simulink model "Lidar_System_FullStateOct25v2"  (Simulink 7.3)
settings: Solver=FixedStepDiscrete  StartTime=0.0  StopTime=inf  FixedStep=0.1  MaxStep=0.2  RelTol=1e-3
undefined symbols (not defined in the file): strel
libraries: dspmtrx3 x28, simulink x11, dspstat3 x10, vipstatistics x6, vipmorphops x6, dspindex x1
(part 1 of 3)
settings Model: Creator=gclayton  LastModifiedBy=wildcat
settings DebuggingCC: InheritedTsInSrcMsg=none
settings RTWCC: SystemTargetFile=rlnx.tlc  GenCodeOnly=on  TemplateMakefile=rlnx_ubuntu.tmf  Description=Linux Real-Time Target  ProcessScript=rlnx_make_rtw_hook
settings RTWCC: CustomInclude=|
  | /usr/local/include/opencv/
  | /usr/local/include/
settings CodeAppCC: GenerateComments=off  SimulinkBlockComments=off
settings STFCustomTargetCC: ModelReferenceCompliant=off  MatFileLogging=on  SystemTargetFile=rlnx.tlc
settings GRTTargetCC: ModelReferenceCompliant=off  ParMdlRefBuildCompliant=off  CompOptLevelCompliant=off  ExtModeMexFile=noextcomm
settings CustomProperty: DataType=string  Value="-lm -ldl /usr/local/lib/libopencv_highgui.so.2.4 /usr/local/lib/libopencv_core.so.2.4 /usr/local/lib/libopencv_imgproc.so.2.4  -lc_urg -lc_urg_connection -lc_urg_system -lphidget21 -llcm"
settings EnumStrPairs: String=PC

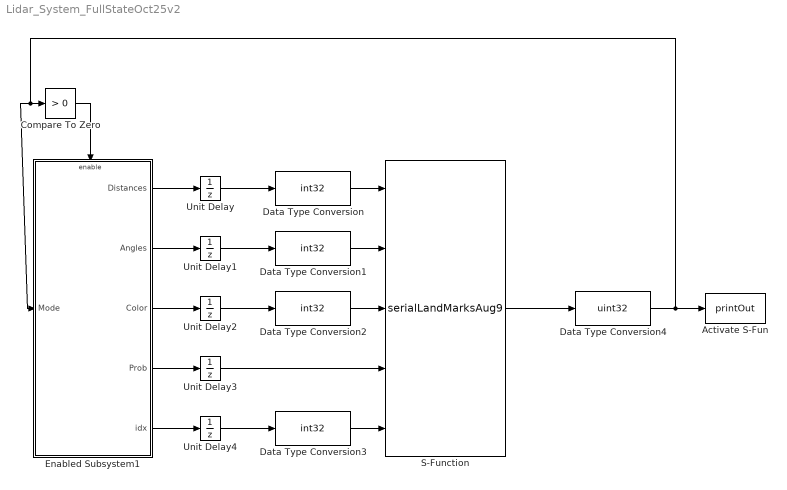
== system Lidar_System_FullStateOct25v2 ==
  Activate S-Fun : S-Function  FunctionName=printOut  EnableBusSupport=off
  Compare To Zero : simulink/Logic and Bit Operations/Compare To Zero  SystemSampleTime=-1  relop=>  LogicOutDataTypeMode=uint8  ZeroCross=off
  Data Type Conversion{,1..3} (4 alike) : DataTypeConversion  OutDataTypeMode=int32  OutDataType=fixdt(1, 16)  OutScaling=2^0  OutDataTypeStr=int32
  Data Type Conversion4 : DataTypeConversion  OutDataTypeMode=uint32  OutDataType=fixdt(1, 16)  OutScaling=2^0  OutDataTypeStr=uint32
  Enabled Subsystem1 : Subsystem  TreatAsAtomicUnit=on
  S-Function : S-Function  FunctionName=serialLandMarksAug9  EnableBusSupport=off
  Unit Delay : UnitDelay  X0=zeros(1,12)  SampleTime=-1
  Unit Delay1 : UnitDelay  X0=zeros(1,12)  SampleTime=-1
  Unit Delay2 : UnitDelay  X0=zeros(4,1)  SampleTime=-1
  Unit Delay3 : UnitDelay  X0=zeros(4,1)  SampleTime=-1
  Unit Delay4 : UnitDelay  X0=zeros(4,1)  SampleTime=-1
  wires:
  Compare To Zero/1 -> Enabled Subsystem1/Enable
  Data Type Conversion4/1 -> Activate S-Fun/1, Compare To Zero/1, Enabled Subsystem1/1(Mode)
  S-Function/1 -> Data Type Conversion4/1
  Enabled Subsystem1/2(Angles) -> Unit Delay1/1
  Enabled Subsystem1/1(Distances) -> Unit Delay/1
  Enabled Subsystem1/3(Color) -> Unit Delay2/1
  Enabled Subsystem1/4(Prob) -> Unit Delay3/1
  Enabled Subsystem1/5(idx) -> Unit Delay4/1
  Unit Delay/1 -> Data Type Conversion/1
  Unit Delay1/1 -> Data Type Conversion1/1
  Unit Delay2/1 -> Data Type Conversion2/1
  Unit Delay4/1 -> Data Type Conversion3/1
  Data Type Conversion/1 -> S-Function/1
  Data Type Conversion1/1 -> S-Function/2
  Data Type Conversion2/1 -> S-Function/3
  Unit Delay3/1 -> S-Function/4
  Data Type Conversion3/1 -> S-Function/5

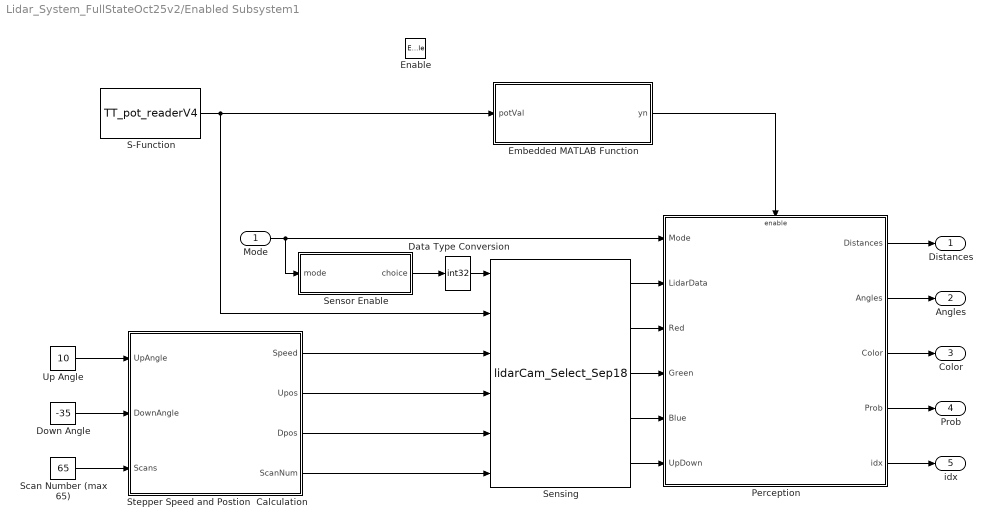
== system Lidar_System_FullStateOct25v2/Enabled Subsystem1 ==
  Mode : Inport  OutDataType=fixdt(1, 16)  OutScaling=2^0
  Enable : EnablePort
  Data Type Conversion : DataTypeConversion  OutDataTypeMode=int32  OutDataType=fixdt(1, 16)  OutScaling=2^0  OutDataTypeStr=int32
  Down Angle : Constant  Value=-35  OutDataType=fixdt(1, 16)  OutScaling=2^0
  Embedded MATLAB Function : Stateflow chart
  Perception : Subsystem  TreatAsAtomicUnit=on
  S-Function : S-Function  FunctionName=TT_pot_readerV4  EnableBusSupport=off
  Scan Number (max 65) : Constant  Value=65  OutDataType=fixdt(1, 16)  OutScaling=2^0
  Sensing : S-Function  FunctionName=lidarCam_Select_Sep18  EnableBusSupport=off
  Sensor Enable : Stateflow chart
  Stepper Speed and Postion  Calculation : Stateflow chart
  Up Angle : Constant  Value=10  OutDataType=fixdt(1, 16)  OutScaling=2^0
  Distances : Outport  OutDataType=fixdt(1, 16)  OutScaling=2^0
  Angles : Outport  Port=2  OutDataType=fixdt(1, 16)  OutScaling=2^0
  Color : Outport  Port=3  OutDataType=fixdt(1, 16)  OutScaling=2^0
  Prob : Outport  Port=4  OutDataType=fixdt(1, 16)  OutScaling=2^0
  idx : Outport  Port=5  OutDataType=fixdt(1, 16)  OutScaling=2^0
  wires:
  Embedded MATLAB Function/1(yn) -> Perception/Enable
  Sensing/1 -> Perception/2(LidarData)
  Sensing/5 -> Perception/6(UpDown)
  Sensing/2 -> Perception/3(Red)
  Sensing/3 -> Perception/4(Green)
  Sensing/4 -> Perception/5(Blue)
  Mode/1 -> Perception/1(Mode), Sensor Enable/1(mode)
  Down Angle/1 -> Stepper Speed and Postion  Calculation/2(DownAngle)
  Up Angle/1 -> Stepper Speed and Postion  Calculation/1(UpAngle)
  Scan Number (max 65)/1 -> Stepper Speed and Postion  Calculation/3(Scans)
  Stepper Speed and Postion  Calculation/1(Speed) -> Sensing/3
  Stepper Speed and Postion  Calculation/2(Upos) -> Sensing/4
  Stepper Speed and Postion  Calculation/3(Dpos) -> Sensing/5
  Stepper Speed and Postion  Calculation/4(ScanNum) -> Sensing/6
  S-Function/1 -> Embedded MATLAB Function/1(potVal), Sensing/2
  Sensor Enable/1(choice) -> Data Type Conversion/1
  Data Type Conversion/1 -> Sensing/1
  Perception/1(Distances) -> Distances/1
  Perception/2(Angles) -> Angles/1
  Perception/3(Color) -> Color/1
  Perception/4(Prob) -> Prob/1
  Perception/5(idx) -> idx/1

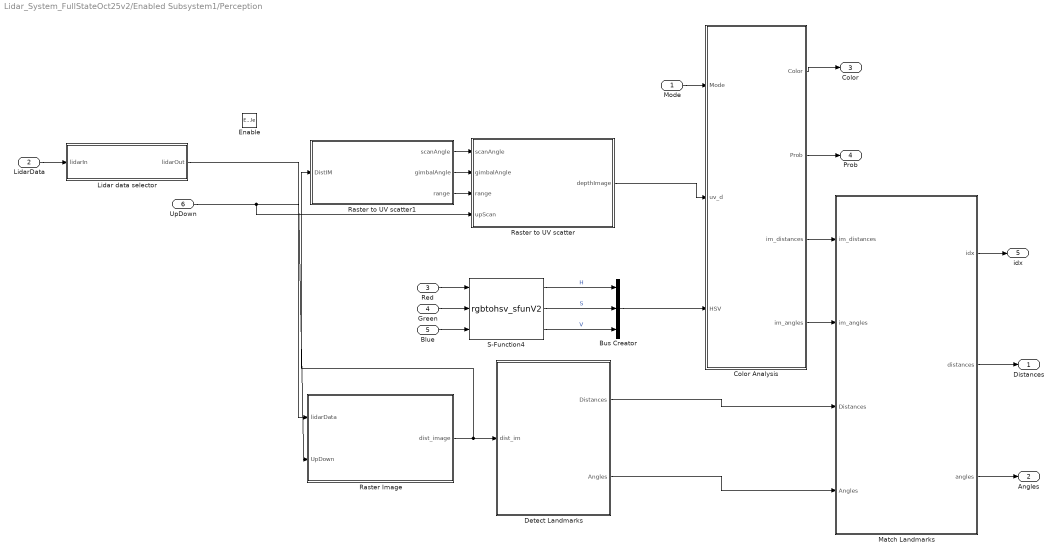
== system Lidar_System_FullStateOct25v2/Enabled Subsystem1/Perception ==
  Mode : Inport  OutDataType=fixdt(1, 16)  OutScaling=2^0
  LidarData : Inport  Port=2  OutDataType=fixdt(1, 16)  OutScaling=2^0
  Red : Inport  Port=3  OutDataType=fixdt(1, 16)  OutScaling=2^0
  Green : Inport  Port=4  OutDataType=fixdt(1, 16)  OutScaling=2^0
  Blue : Inport  Port=5  OutDataType=fixdt(1, 16)  OutScaling=2^0
  UpDown : Inport  Port=6  OutDataType=fixdt(1, 16)  OutScaling=2^0
  Enable : EnablePort
  Bus Creator : BusCreator  Inputs=3
  Color Analysis : Subsystem
  Detect Landmarks : Subsystem
  Lidar data selector : Stateflow chart
  Match Landmarks : Stateflow chart
  Raster Image : Stateflow chart
  Raster to UV scatter : Stateflow chart
  Raster to UV scatter1 : Stateflow chart
  S-Function4 : S-Function  FunctionName=rgbtohsv_sfunV2  EnableBusSupport=off
  Distances : Outport  OutDataType=fixdt(1, 16)  OutScaling=2^0
  Angles : Outport  Port=2  OutDataType=fixdt(1, 16)  OutScaling=2^0
  Color : Outport  Port=3  OutDataType=fixdt(1, 16)  OutScaling=2^0
  Prob : Outport  Port=4  OutDataType=fixdt(1, 16)  OutScaling=2^0
  idx : Outport  Port=5  OutDataType=fixdt(1, 16)  OutScaling=2^0
  wires:
  Lidar data selector/1(lidarOut) -> Raster Image/1(lidarData)
  UpDown/1 -> Raster Image/2(UpDown), Raster to UV scatter/4(upScan)
  Red/1 -> S-Function4/1
  Green/1 -> S-Function4/2
  Blue/1 -> S-Function4/3
  LidarData/1 -> Lidar data selector/1(lidarIn)
  S-Function4/1 -> Bus Creator/1  "H"
  S-Function4/2 -> Bus Creator/2  "S"
  S-Function4/3 -> Bus Creator/3  "V"
  Bus Creator/1 -> Color Analysis/3(HSV)
  Raster to UV scatter/1(depthImage) -> Color Analysis/2(uv_d)
  Mode/1 -> Color Analysis/1(Mode)
  Color Analysis/2(Prob) -> Prob/1
  Color Analysis/1(Color) -> Color/1
  Color Analysis/3(im_distances) -> Match Landmarks/1(im_distances)
  Color Analysis/4(im_angles) -> Match Landmarks/2(im_angles)
  Detect Landmarks/1(Distances) -> Match Landmarks/3(Distances)
  Detect Landmarks/2(Angles) -> Match Landmarks/4(Angles)
  Raster Image/1(dist_image) -> Detect Landmarks/1(dist_im), Raster to UV scatter1/1(DistIM)
  Raster to UV scatter1/1(scanAngle) -> Raster to UV scatter/1(scanAngle)
  Raster to UV scatter1/2(gimbalAngle) -> Raster to UV scatter/2(gimbalAngle)
  Raster to UV scatter1/3(range) -> Raster to UV scatter/3(range)
  Match Landmarks/1(idx) -> idx/1
  Match Landmarks/2(distances) -> Distances/1
  Match Landmarks/3(angles) -> Angles/1

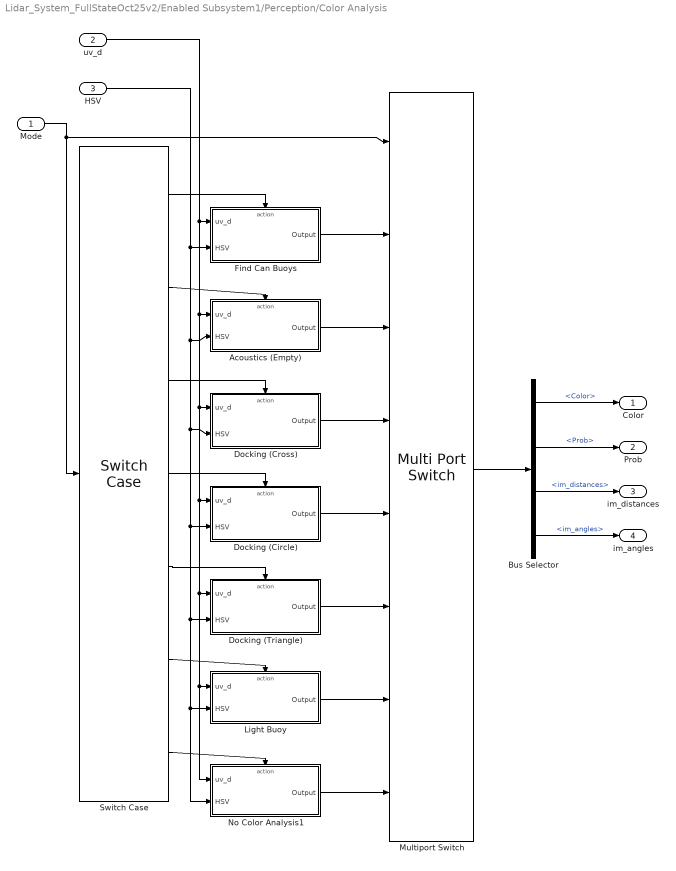
== system Lidar_System_FullStateOct25v2/Enabled Subsystem1/Perception/Color Analysis ==
  Mode : Inport  OutDataType=fixdt(1, 16)  OutScaling=2^0
  uv_d : Inport  Port=2  OutDataType=fixdt(1, 16)  OutScaling=2^0
  HSV : Inport  Port=3  OutDataType=fixdt(1, 16)  OutScaling=2^0
  Acoustics (Empty) : Subsystem  TreatAsAtomicUnit=on
  Bus Selector : BusSelector  OutputSignals=Color,Prob,im_distances,im_angles
  Docking (Circle) : Subsystem  TreatAsAtomicUnit=on
  Docking (Cross) : Subsystem  TreatAsAtomicUnit=on
  Docking (Triangle) : Subsystem  TreatAsAtomicUnit=on
  Find Can Buoys : Subsystem  TreatAsAtomicUnit=on
  Light Buoy : Subsystem  TreatAsAtomicUnit=on
  Multiport Switch : MultiPortSwitch  Inputs=7  OutDataType=fixdt(1, 16)  OutScaling=2^0
  No Color Analysis1 : Subsystem  TreatAsAtomicUnit=on
  Switch Case : SwitchCase  CaseConditions={1,2,3,4,5,6}
  Color : Outport  OutDataType=fixdt(1, 16)  OutScaling=2^0
  Prob : Outport  Port=2  OutDataType=fixdt(1, 16)  OutScaling=2^0
  im_distances : Outport  Port=3  OutDataType=fixdt(1, 16)  OutScaling=2^0
  im_angles : Outport  Port=4  OutDataType=fixdt(1, 16)  OutScaling=2^0
  wires:
  Switch Case/1 -> Find Can Buoys/Action
  Mode/1 -> Switch Case/1, Multiport Switch/1
  Switch Case/2 -> Acoustics (Empty)/Action
  Switch Case/3 -> Docking (Cross)/Action
  Find Can Buoys/1(Output) -> Multiport Switch/2
  Docking (Cross)/1(Output) -> Multiport Switch/4
  Docking (Circle)/1(Output) -> Multiport Switch/5
  uv_d/1 -> Docking (Cross)/1(uv_d), Docking (Circle)/1(uv_d), Docking (Triangle)/1(uv_d), Light Buoy/1(uv_d), No Color Analysis1/1(uv_d), Acoustics (Empty)/1(uv_d), Find Can Buoys/1(uv_d)
  HSV/1 -> Docking (Cross)/2(HSV), Docking (Circle)/2(HSV), Docking (Triangle)/2(HSV), Light Buoy/2(HSV), No Color Analysis1/2(HSV), Acoustics (Empty)/2(HSV), Find Can Buoys/2(HSV)
  Acoustics (Empty)/1(Output) -> Multiport Switch/3
  Bus Selector/1 -> Color/1  "<Color>"
  Bus Selector/2 -> Prob/1  "<Prob>"
  Bus Selector/3 -> im_distances/1  "<im_distances>"
  Bus Selector/4 -> im_angles/1  "<im_angles>"
  Switch Case/4 -> Docking (Circle)/Action
  Switch Case/7 -> No Color Analysis1/Action
  Switch Case/5 -> Docking (Triangle)/Action
  Switch Case/6 -> Light Buoy/Action
  Docking (Triangle)/1(Output) -> Multiport Switch/6
  Light Buoy/1(Output) -> Multiport Switch/7
  No Color Analysis1/1(Output) -> Multiport Switch/8
  Multiport Switch/1 -> Bus Selector/1

== system Lidar_System_FullStateOct25v2/Enabled Subsystem1/Perception/Detect Landmarks ==
  dist_im : Inport  OutDataType=fixdt(1, 16)  OutScaling=2^0
  Blob Analysis : vipstatistics/Blob Analysis  DialogController=vipDDGCreate  DialogControllerArgs=DataTag15  area=off  centroid=on  bBox=on  majorAxis=off  minorAxis=off  angle=off  eccentricity=off  equivDiameterSq=off  extent=off  perimeter=off  maxBlobs=12  warnIfNumBlobsExceeded=on  isCount=off  useMinArea=on  minArea=30  useMaxArea=off  maxArea=intmax('uint32')  excludeBorderBlob=on  outDT=double  isOutVarDim=off  isFill=on  fillValues=-1  conn=8  isLabel=off  outputMode=Binary point scaling  outputWordLength=32  outputFracLength=16  firstCoeffMode=Binary point scaling  firstCoeffWordLength=16  firstCoeffFracLength=14  secondCoeffMode=Binary point scaling  secondCoeffWordLength=32  secondCoeffFracLength=16  accumMode=Binary point scaling  accumWordLength=32  accumFracLength=0  prodOutputMode=Binary point scaling  prodOutputWordLength=32  prodOutputFracLength=16  roundingMode=Floor  overflowMode=off
  Closing : vipmorphops/Closing  nhoodsrc=Specify via dialog  strel=strel('rectangle',[5 7])
  Embedded MATLAB Function1 : Stateflow chart
  Logical Operator : Logic  AllPortsSameDT=off  OutDataTypeMode=boolean  LogicDataType=fixdt(0, 8)  OutDataTypeStr=boolean
  Max Thresh : simulink/Logic and Bit Operations/Compare To Constant  SystemSampleTime=-1  relop=<=  const=10000  LogicOutDataTypeMode=boolean  ZeroCross=off
  Min Thresh (removes pontoons) : simulink/Logic and Bit Operations/Compare To Constant  SystemSampleTime=-1  relop=>  const=5000  LogicOutDataTypeMode=boolean  ZeroCross=off
  Distances : Outport  OutDataType=fixdt(1, 16)  OutScaling=2^0
  Angles : Outport  Port=2  OutDataType=fixdt(1, 16)  OutScaling=2^0
  wires:
  Max Thresh/1 -> Logical Operator/1
  Min Thresh (removes pontoons)/1 -> Logical Operator/2
  dist_im/1 -> Max Thresh/1, Min Thresh (removes pontoons)/1, Embedded MATLAB Function1/4(dist_im)
  Embedded MATLAB Function1/1(Distances) -> Distances/1
  Embedded MATLAB Function1/2(Angles) -> Angles/1
  Logical Operator/1 -> Closing/1, Embedded MATLAB Function1/3(BW)
  Closing/1 -> Blob Analysis/1
  Blob Analysis/1 -> Embedded MATLAB Function1/1(centroid)
  Blob Analysis/2 -> Embedded MATLAB Function1/2(bbox)

== system Lidar_System_FullStateOct25v2/Enabled Subsystem1/Perception/Color Analysis/Acoustics (Empty) ==
  uv_d : Inport  OutDataType=fixdt(1, 16)  OutScaling=2^0
  HSV : Inport  Port=2  OutDataType=fixdt(1, 16)  OutScaling=2^0
  Action Port : ActionPort  ActionType=case
  Bus Creator : BusCreator
  Constant{,1..3} (4 alike) : Constant  Value=zeros(4,1)  OutDataType=fixdt(1, 16)  OutScaling=2^0
  Terminator : Terminator
  Terminator1 : Terminator
  Output : Outport  OutDataType=fixdt(1, 16)  OutScaling=2^0
  wires:
  uv_d/1 -> Terminator/1
  HSV/1 -> Terminator1/1
  Bus Creator/1 -> Output/1
  Constant3/1 -> Bus Creator/4  "im_angles"
  Constant2/1 -> Bus Creator/3  "im_distances"
  Constant1/1 -> Bus Creator/2  "Prob"
  Constant/1 -> Bus Creator/1  "Color"

== system Lidar_System_FullStateOct25v2/Enabled Subsystem1/Perception/Color Analysis/Docking (Circle) ==
  uv_d : Inport  OutDataType=fixdt(1, 16)  OutScaling=2^0
  HSV : Inport  Port=2  OutDataType=fixdt(1, 16)  OutScaling=2^0
  Action Port : ActionPort  ActionType=case
  Bus Creator : BusCreator
  Bus Selector : BusSelector  OutputSignals=H,S,V
  Constant : Constant  Value=zeros(4,1)  OutDataType=fixdt(1, 16)  OutScaling=2^0
  Constant1 : Constant  Value=zeros(4,1)  OutDataType=fixdt(1, 16)  OutScaling=2^0
  Constant4 : Constant  Value=2  OutDataType=fixdt(1, 16)  OutScaling=2^0
  Docking1 : Subsystem
  Output : Outport  OutDataType=fixdt(1, 16)  OutScaling=2^0
  wires:
  Constant/1 -> Bus Creator/1  "Color"
  Constant1/1 -> Bus Creator/2  "Prob"
  Docking1/1(Distances) -> Bus Creator/3  "im_distances"
  Docking1/2(Angles) -> Bus Creator/4  "im_angles"
  Bus Creator/1 -> Output/1
  Constant4/1 -> Docking1/1(Target)
  Bus Selector/1 -> Docking1/2(H)  "<H>"
  Bus Selector/2 -> Docking1/3(S)  "<S>"
  Bus Selector/3 -> Docking1/4(V)  "<V>"
  HSV/1 -> Bus Selector/1
  uv_d/1 -> Docking1/5(uv_d)

== system Lidar_System_FullStateOct25v2/Enabled Subsystem1/Perception/Color Analysis/Docking (Cross) ==
  uv_d : Inport  OutDataType=fixdt(1, 16)  OutScaling=2^0
  HSV : Inport  Port=2  OutDataType=fixdt(1, 16)  OutScaling=2^0
  Action Port : ActionPort  ActionType=case
  Bus Creator : BusCreator
  Bus Selector : BusSelector  OutputSignals=H,S,V
  Constant : Constant  Value=zeros(4,1)  OutDataType=fixdt(1, 16)  OutScaling=2^0
  Constant1 : Constant  Value=zeros(4,1)  OutDataType=fixdt(1, 16)  OutScaling=2^0
  Constant4 : Constant  OutDataType=fixdt(1, 16)  OutScaling=2^0
  Docking1 : Subsystem
  Output : Outport  OutDataType=fixdt(1, 16)  OutScaling=2^0
  wires:
  uv_d/1 -> Docking1/5(uv_d)
  HSV/1 -> Bus Selector/1
  Bus Selector/3 -> Docking1/4(V)  "<V>"
  Bus Selector/2 -> Docking1/3(S)  "<S>"
  Bus Selector/1 -> Docking1/2(H)  "<H>"
  Constant4/1 -> Docking1/1(Target)
  Bus Creator/1 -> Output/1
  Docking1/2(Angles) -> Bus Creator/4  "im_angles"
  Docking1/1(Distances) -> Bus Creator/3  "im_distances"
  Constant1/1 -> Bus Creator/2  "Prob"
  Constant/1 -> Bus Creator/1  "Color"

== system Lidar_System_FullStateOct25v2/Enabled Subsystem1/Perception/Color Analysis/Docking (Triangle) ==
  uv_d : Inport  OutDataType=fixdt(1, 16)  OutScaling=2^0
  HSV : Inport  Port=2  OutDataType=fixdt(1, 16)  OutScaling=2^0
  Action Port : ActionPort  ActionType=case
  Bus Creator : BusCreator
  Bus Selector : BusSelector  OutputSignals=H,S,V
  Constant : Constant  Value=zeros(4,1)  OutDataType=fixdt(1, 16)  OutScaling=2^0
  Constant1 : Constant  Value=zeros(4,1)  OutDataType=fixdt(1, 16)  OutScaling=2^0
  Constant4 : Constant  Value=3  OutDataType=fixdt(1, 16)  OutScaling=2^0
  Docking1 : Subsystem
  Output : Outport  OutDataType=fixdt(1, 16)  OutScaling=2^0
  wires:
  uv_d/1 -> Docking1/5(uv_d)
  HSV/1 -> Bus Selector/1
  Bus Selector/3 -> Docking1/4(V)  "<V>"
  Bus Selector/2 -> Docking1/3(S)  "<S>"
  Bus Selector/1 -> Docking1/2(H)  "<H>"
  Constant4/1 -> Docking1/1(Target)
  Bus Creator/1 -> Output/1
  Docking1/2(Angles) -> Bus Creator/4  "im_angles"
  Docking1/1(Distances) -> Bus Creator/3  "im_distances"
  Constant1/1 -> Bus Creator/2  "Prob"
  Constant/1 -> Bus Creator/1  "Color"

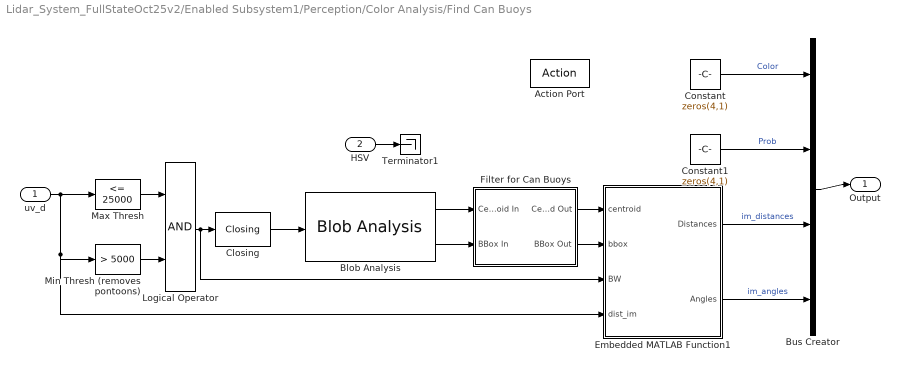
== system Lidar_System_FullStateOct25v2/Enabled Subsystem1/Perception/Color Analysis/Find Can Buoys ==
  uv_d : Inport  OutDataType=fixdt(1, 16)  OutScaling=2^0
  HSV : Inport  Port=2  OutDataType=fixdt(1, 16)  OutScaling=2^0
  Action Port : ActionPort  ActionType=case
  Blob Analysis : vipstatistics/Blob Analysis  DialogController=vipDDGCreate  DialogControllerArgs=DataTag12  area=off  centroid=on  bBox=on  majorAxis=off  minorAxis=off  angle=off  eccentricity=off  equivDiameterSq=off  extent=off  perimeter=off  maxBlobs=12  warnIfNumBlobsExceeded=on  isCount=off  useMinArea=on  minArea=30  useMaxArea=off  maxArea=intmax('uint32')  excludeBorderBlob=on  outDT=double  isOutVarDim=off  isFill=on  fillValues=-1  conn=8  isLabel=off  outputMode=Binary point scaling  outputWordLength=32  outputFracLength=16  firstCoeffMode=Binary point scaling  firstCoeffWordLength=16  firstCoeffFracLength=14  secondCoeffMode=Binary point scaling  secondCoeffWordLength=32  secondCoeffFracLength=16  accumMode=Binary point scaling  accumWordLength=32  accumFracLength=0  prodOutputMode=Binary point scaling  prodOutputWordLength=32  prodOutputFracLength=16  roundingMode=Floor  overflowMode=off
  Bus Creator : BusCreator
  Closing : vipmorphops/Closing  nhoodsrc=Specify via dialog  strel=strel('rectangle',[5 7])
  Constant : Constant  Value=zeros(4,1)  OutDataType=fixdt(1, 16)  OutScaling=2^0
  Constant1 : Constant  Value=zeros(4,1)  OutDataType=fixdt(1, 16)  OutScaling=2^0
  Embedded MATLAB Function1 : Stateflow chart
  Filter for Can Buoys : Subsystem
  Logical Operator : Logic  AllPortsSameDT=off  OutDataTypeMode=boolean  LogicDataType=fixdt(0, 8)  OutDataTypeStr=boolean
  Max Thresh : simulink/Logic and Bit Operations/Compare To Constant  SystemSampleTime=-1  relop=<=  const=25000  LogicOutDataTypeMode=boolean  ZeroCross=off
  Min Thresh (removes pontoons) : simulink/Logic and Bit Operations/Compare To Constant  SystemSampleTime=-1  relop=>  const=5000  LogicOutDataTypeMode=boolean  ZeroCross=off
  Terminator1 : Terminator
  Output : Outport  OutDataType=fixdt(1, 16)  OutScaling=2^0
  wires:
  Constant/1 -> Bus Creator/1  "Color"
  Constant1/1 -> Bus Creator/2  "Prob"
  Embedded MATLAB Function1/1(Distances) -> Bus Creator/3  "im_distances"
  Embedded MATLAB Function1/2(Angles) -> Bus Creator/4  "im_angles"
  Bus Creator/1 -> Output/1
  HSV/1 -> Terminator1/1
  Max Thresh/1 -> Logical Operator/1
  Min Thresh (removes pontoons)/1 -> Logical Operator/2
  Logical Operator/1 -> Closing/1, Embedded MATLAB Function1/3(BW)
  Closing/1 -> Blob Analysis/1
  uv_d/1 -> Max Thresh/1, Min Thresh (removes pontoons)/1, Embedded MATLAB Function1/4(dist_im)
  Blob Analysis/1 -> Filter for Can Buoys/1(Centroid In)
  Blob Analysis/2 -> Filter for Can Buoys/2(BBox In)
  Filter for Can Buoys/1(Centroid Out) -> Embedded MATLAB Function1/1(centroid)
  Filter for Can Buoys/2(BBox Out) -> Embedded MATLAB Function1/2(bbox)

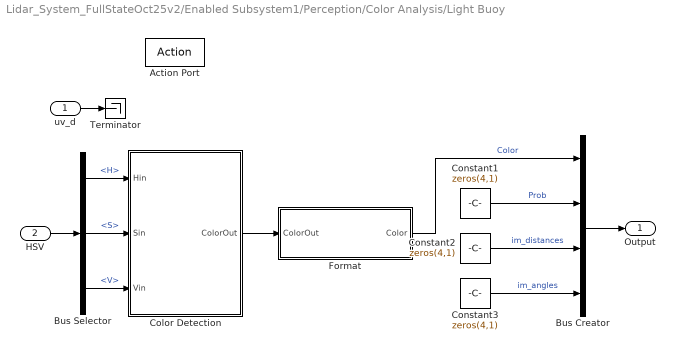
== system Lidar_System_FullStateOct25v2/Enabled Subsystem1/Perception/Color Analysis/Light Buoy ==
  uv_d : Inport  OutDataType=fixdt(1, 16)  OutScaling=2^0
  HSV : Inport  Port=2  OutDataType=fixdt(1, 16)  OutScaling=2^0
  Action Port : ActionPort  ActionType=case
  Bus Creator : BusCreator
  Bus Selector : BusSelector  OutputSignals=H,S,V
  Color Detection : Subsystem
  Constant1 : Constant  Value=zeros(4,1)  OutDataType=fixdt(1, 16)  OutScaling=2^0
  Constant2 : Constant  Value=zeros(4,1)  OutDataType=fixdt(1, 16)  OutScaling=2^0
  Constant3 : Constant  Value=zeros(4,1)  OutDataType=fixdt(1, 16)  OutScaling=2^0
  Format : Stateflow chart
  Terminator : Terminator
  Output : Outport  OutDataType=fixdt(1, 16)  OutScaling=2^0
  wires:
  Color Detection/1(ColorOut) -> Format/1(ColorOut)
  Bus Selector/3 -> Color Detection/3(Vin)  "<V>"
  Bus Selector/2 -> Color Detection/2(Sin)  "<S>"
  Bus Selector/1 -> Color Detection/1(Hin)  "<H>"
  HSV/1 -> Bus Selector/1
  uv_d/1 -> Terminator/1
  Bus Creator/1 -> Output/1
  Constant3/1 -> Bus Creator/4  "im_angles"
  Constant2/1 -> Bus Creator/3  "im_distances"
  Constant1/1 -> Bus Creator/2  "Prob"
  Format/1(Color) -> Bus Creator/1  "Color"

== system Lidar_System_FullStateOct25v2/Enabled Subsystem1/Perception/Color Analysis/No Color Analysis1 ==
  uv_d : Inport  OutDataType=fixdt(1, 16)  OutScaling=2^0
  HSV : Inport  Port=2  OutDataType=fixdt(1, 16)  OutScaling=2^0
  Action Port : ActionPort  ActionType=default
  Bus Creator : BusCreator
  Constant{,1..3} (4 alike) : Constant  Value=zeros(4,1)  OutDataType=fixdt(1, 16)  OutScaling=2^0
  Terminator : Terminator
  Terminator1 : Terminator
  Output : Outport  OutDataType=fixdt(1, 16)  OutScaling=2^0
  wires:
  Constant/1 -> Bus Creator/1  "Color"
  Constant1/1 -> Bus Creator/2  "Prob"
  Constant2/1 -> Bus Creator/3  "im_distances"
  Constant3/1 -> Bus Creator/4  "im_angles"
  Bus Creator/1 -> Output/1
  HSV/1 -> Terminator1/1
  uv_d/1 -> Terminator/1

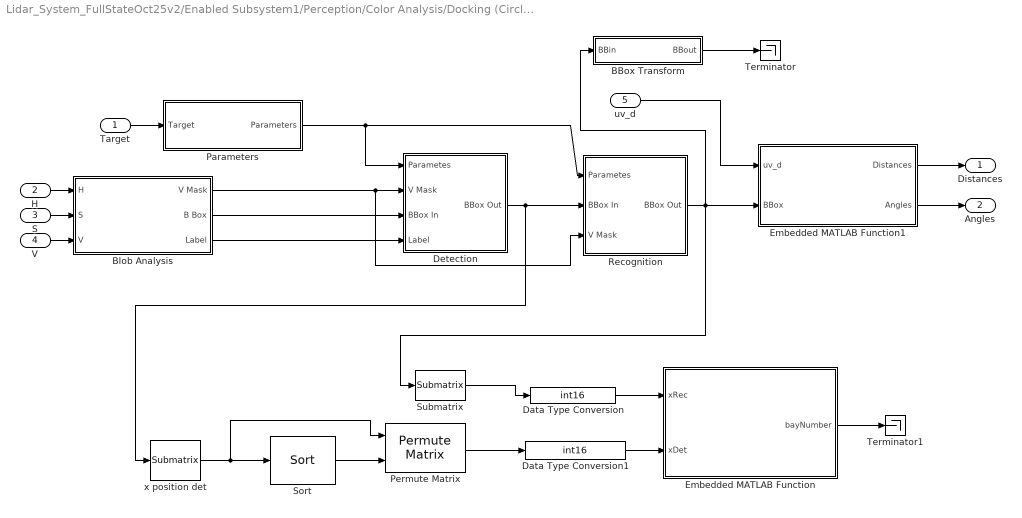
== system Lidar_System_FullStateOct25v2/Enabled Subsystem1/Perception/Color Analysis/Docking (Circle)/Docking1 ==
  Target : Inport
  H : Inport  Port=2
  S : Inport  Port=3
  V : Inport  Port=4
  uv_d : Inport  Port=5
  BBox Transform : Stateflow chart
  Blob Analysis : Subsystem
  Data Type Conversion : DataTypeConversion  OutDataTypeMode=int16  OutDataType=fixdt(1, 16)  OutScaling=2^0  OutDataTypeStr=int16
  Data Type Conversion1 : DataTypeConversion  OutDataTypeMode=int16  OutDataType=fixdt(1, 16)  OutScaling=2^0  OutDataTypeStr=int16
  Detection : Subsystem
  Embedded MATLAB Function : Stateflow chart
  Embedded MATLAB Function1 : Stateflow chart
  Parameters : Subsystem
  Permute Matrix : dspmtrx3/Permute Matrix  mode=Rows  ZeroOneIdxMode=One-based  errmode=Clip index  checkDims=off
  Recognition : Subsystem
  Sort : dspstat3/Sort  DialogController=dspDDGCreate  DialogControllerArgs=DataTag3  otype=Index  dir=Ascending  sortAlg=Quick sort  roundingMode=Floor  overflowMode=off
  Submatrix : dspmtrx3/Submatrix  RowSpan=Range of rows  RowStartMode=First  RowStartIndex=1  RowEndMode=Last  RowEndIndex=1  ColSpan=One column  ColStartMode=First  ColStartIndex=1  ColEndMode=Last  ColEndIndex=1
  Terminator : Terminator
  Terminator1 : Terminator
  x position det : dspmtrx3/Submatrix  RowSpan=Range of rows  RowStartMode=First  RowStartIndex=1  RowEndMode=Last  RowEndIndex=1  ColSpan=One column  ColStartMode=First  ColStartIndex=1  ColEndMode=Last  ColEndIndex=1
  Distances : Outport
  Angles : Outport  Port=2
  wires:
  Parameters/1(Parameters) -> Detection/1(Parametes), Recognition/1(Parametes)
  Blob Analysis/1(V Mask) -> Detection/2(V Mask), Recognition/3(V Mask)
  Blob Analysis/2(B Box) -> Detection/3(BBox In)
  Blob Analysis/3(Label) -> Detection/4(Label)
  Detection/1(BBox Out) -> Recognition/2(BBox In), x position det/1
  x position det/1 -> Sort/1, Permute Matrix/1
  Sort/1 -> Permute Matrix/2
  Submatrix/1 -> Data Type Conversion/1
  Permute Matrix/1 -> Data Type Conversion1/1
  Data Type Conversion/1 -> Embedded MATLAB Function/1(xRec)
  Data Type Conversion1/1 -> Embedded MATLAB Function/2(xDet)
  Recognition/1(BBox Out) -> Submatrix/1, Embedded MATLAB Function1/2(BBox), BBox Transform/1(BBin)
  Embedded MATLAB Function/1(bayNumber) -> Terminator1/1
  uv_d/1 -> Embedded MATLAB Function1/1(uv_d)
  Embedded MATLAB Function1/1(Distances) -> Distances/1
  H/1 -> Blob Analysis/1(H)
  S/1 -> Blob Analysis/2(S)
  V/1 -> Blob Analysis/3(V)
  Target/1 -> Parameters/1(Target)
  BBox Transform/1(BBout) -> Terminator/1
  Embedded MATLAB Function1/2(Angles) -> Angles/1

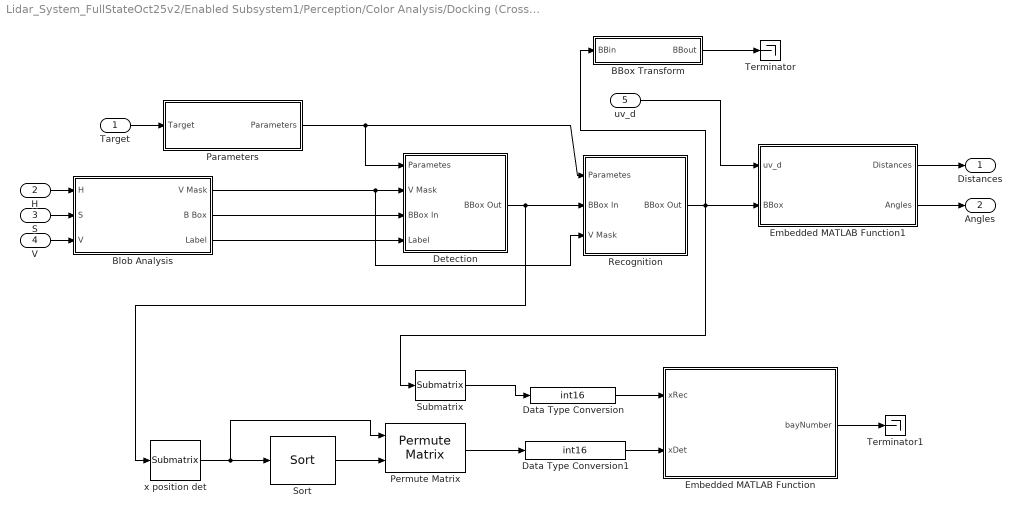
== system Lidar_System_FullStateOct25v2/Enabled Subsystem1/Perception/Color Analysis/Docking (Cross)/Docking1 ==
  Target : Inport
  H : Inport  Port=2
  S : Inport  Port=3
  V : Inport  Port=4
  uv_d : Inport  Port=5
  BBox Transform : Stateflow chart
  Blob Analysis : Subsystem
  Data Type Conversion : DataTypeConversion  OutDataTypeMode=int16  OutDataType=fixdt(1, 16)  OutScaling=2^0  OutDataTypeStr=int16
  Data Type Conversion1 : DataTypeConversion  OutDataTypeMode=int16  OutDataType=fixdt(1, 16)  OutScaling=2^0  OutDataTypeStr=int16
  Detection : Subsystem
  Embedded MATLAB Function : Stateflow chart
  Embedded MATLAB Function1 : Stateflow chart
  Parameters : Subsystem
  Permute Matrix : dspmtrx3/Permute Matrix  mode=Rows  ZeroOneIdxMode=One-based  errmode=Clip index  checkDims=off
  Recognition : Subsystem
  Sort : dspstat3/Sort  DialogController=dspDDGCreate  DialogControllerArgs=DataTag7  otype=Index  dir=Ascending  sortAlg=Quick sort  roundingMode=Floor  overflowMode=off
  Submatrix : dspmtrx3/Submatrix  RowSpan=Range of rows  RowStartMode=First  RowStartIndex=1  RowEndMode=Last  RowEndIndex=1  ColSpan=One column  ColStartMode=First  ColStartIndex=1  ColEndMode=Last  ColEndIndex=1
  Terminator : Terminator
  Terminator1 : Terminator
  x position det : dspmtrx3/Submatrix  RowSpan=Range of rows  RowStartMode=First  RowStartIndex=1  RowEndMode=Last  RowEndIndex=1  ColSpan=One column  ColStartMode=First  ColStartIndex=1  ColEndMode=Last  ColEndIndex=1
  Distances : Outport
  Angles : Outport  Port=2
  wires:
  Embedded MATLAB Function1/2(Angles) -> Angles/1
  BBox Transform/1(BBout) -> Terminator/1
  Target/1 -> Parameters/1(Target)
  V/1 -> Blob Analysis/3(V)
  S/1 -> Blob Analysis/2(S)
  H/1 -> Blob Analysis/1(H)
  Embedded MATLAB Function1/1(Distances) -> Distances/1
  uv_d/1 -> Embedded MATLAB Function1/1(uv_d)
  Embedded MATLAB Function/1(bayNumber) -> Terminator1/1
  Recognition/1(BBox Out) -> BBox Transform/1(BBin), Embedded MATLAB Function1/2(BBox), Submatrix/1
  Data Type Conversion1/1 -> Embedded MATLAB Function/2(xDet)
  Data Type Conversion/1 -> Embedded MATLAB Function/1(xRec)
  Permute Matrix/1 -> Data Type Conversion1/1
  Submatrix/1 -> Data Type Conversion/1
  Sort/1 -> Permute Matrix/2
  x position det/1 -> Permute Matrix/1, Sort/1
  Detection/1(BBox Out) -> x position det/1, Recognition/2(BBox In)
  Blob Analysis/3(Label) -> Detection/4(Label)
  Blob Analysis/2(B Box) -> Detection/3(BBox In)
  Blob Analysis/1(V Mask) -> Recognition/3(V Mask), Detection/2(V Mask)
  Parameters/1(Parameters) -> Recognition/1(Parametes), Detection/1(Parametes)

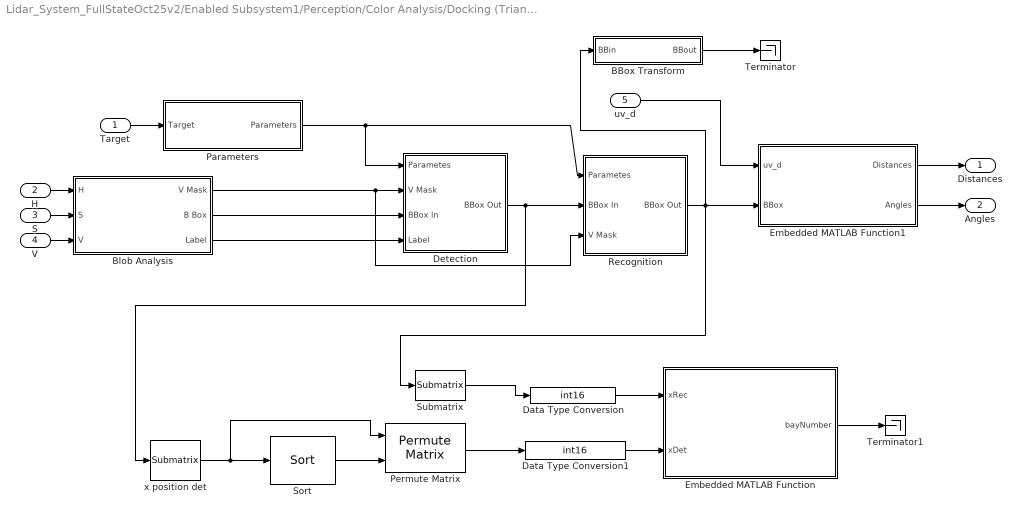
== system Lidar_System_FullStateOct25v2/Enabled Subsystem1/Perception/Color Analysis/Docking (Triangle)/Docking1 ==
  Target : Inport
  H : Inport  Port=2
  S : Inport  Port=3
  V : Inport  Port=4
  uv_d : Inport  Port=5
  BBox Transform : Stateflow chart
  Blob Analysis : Subsystem
  Data Type Conversion : DataTypeConversion  OutDataTypeMode=int16  OutDataType=fixdt(1, 16)  OutScaling=2^0  OutDataTypeStr=int16
  Data Type Conversion1 : DataTypeConversion  OutDataTypeMode=int16  OutDataType=fixdt(1, 16)  OutScaling=2^0  OutDataTypeStr=int16
  Detection : Subsystem
  Embedded MATLAB Function : Stateflow chart
  Embedded MATLAB Function1 : Stateflow chart
  Parameters : Subsystem
  Permute Matrix : dspmtrx3/Permute Matrix  mode=Rows  ZeroOneIdxMode=One-based  errmode=Clip index  checkDims=off
  Recognition : Subsystem
  Sort : dspstat3/Sort  DialogController=dspDDGCreate  DialogControllerArgs=DataTag11  otype=Index  dir=Ascending  sortAlg=Quick sort  roundingMode=Floor  overflowMode=off
  Submatrix : dspmtrx3/Submatrix  RowSpan=Range of rows  RowStartMode=First  RowStartIndex=1  RowEndMode=Last  RowEndIndex=1  ColSpan=One column  ColStartMode=First  ColStartIndex=1  ColEndMode=Last  ColEndIndex=1
  Terminator : Terminator
  Terminator1 : Terminator
  x position det : dspmtrx3/Submatrix  RowSpan=Range of rows  RowStartMode=First  RowStartIndex=1  RowEndMode=Last  RowEndIndex=1  ColSpan=One column  ColStartMode=First  ColStartIndex=1  ColEndMode=Last  ColEndIndex=1
  Distances : Outport
  Angles : Outport  Port=2
  wires:
  Embedded MATLAB Function1/2(Angles) -> Angles/1
  BBox Transform/1(BBout) -> Terminator/1
  Target/1 -> Parameters/1(Target)
  V/1 -> Blob Analysis/3(V)
  S/1 -> Blob Analysis/2(S)
  H/1 -> Blob Analysis/1(H)
  Embedded MATLAB Function1/1(Distances) -> Distances/1
  uv_d/1 -> Embedded MATLAB Function1/1(uv_d)
  Embedded MATLAB Function/1(bayNumber) -> Terminator1/1
  Recognition/1(BBox Out) -> BBox Transform/1(BBin), Embedded MATLAB Function1/2(BBox), Submatrix/1
  Data Type Conversion1/1 -> Embedded MATLAB Function/2(xDet)
  Data Type Conversion/1 -> Embedded MATLAB Function/1(xRec)
  Permute Matrix/1 -> Data Type Conversion1/1
  Submatrix/1 -> Data Type Conversion/1
  Sort/1 -> Permute Matrix/2
  x position det/1 -> Permute Matrix/1, Sort/1
  Detection/1(BBox Out) -> x position det/1, Recognition/2(BBox In)
  Blob Analysis/3(Label) -> Detection/4(Label)
  Blob Analysis/2(B Box) -> Detection/3(BBox In)
  Blob Analysis/1(V Mask) -> Recognition/3(V Mask), Detection/2(V Mask)
  Parameters/1(Parameters) -> Recognition/1(Parametes), Detection/1(Parametes)

== system Lidar_System_FullStateOct25v2/Enabled Subsystem1/Perception/Color Analysis/Find Can Buoys/Filter for Can Buoys ==
  Centroid In : Inport  OutDataType=fixdt(1, 16)  OutScaling=2^0
  BBox In : Inport  Port=2  OutDataType=fixdt(1, 16)  OutScaling=2^0
  Compare To Constant : simulink/Logic and Bit Operations/Compare To Constant  SystemSampleTime=-1  relop=<=  const=0.5  LogicOutDataTypeMode=uint8  ZeroCross=off
  Divide : Product  Inputs=*/  OutDataType=fixdt(1, 16)  OutScaling=2^-10
  Height : dspmtrx3/Submatrix  RowSpan=One row  RowStartMode=Index  RowStartIndex=4  RowEndMode=Last  RowEndIndex=1  ColSpan=All columns  ColStartMode=First  ColStartIndex=1  ColEndMode=Last  ColEndIndex=1
  Variable Selector : dspindex/Variable Selector  NumInputs=2  rowsOrCols=Columns  IdxMode=Variable  Elements=[1 3]  ZerOneIdxMode=Zero-based  errmode=Clip Index  FillMode=on  FillValues=-1
  Width : dspmtrx3/Submatrix  RowSpan=One row  RowStartMode=Index  RowStartIndex=3  RowEndMode=Last  RowEndIndex=1  ColSpan=All columns  ColStartMode=First  ColStartIndex=1  ColEndMode=Last  ColEndIndex=1
  Centroid Out : Outport  OutDataType=fixdt(1, 16)  OutScaling=2^0
  BBox Out : Outport  Port=2  OutDataType=fixdt(1, 16)  OutScaling=2^0
  wires:
  Centroid In/1 -> Variable Selector/1
  BBox In/1 -> Width/1, Height/1, Variable Selector/2
  Width/1 -> Divide/1
  Height/1 -> Divide/2
  Divide/1 -> Compare To Constant/1
  Compare To Constant/1 -> Variable Selector/3
  Variable Selector/2 -> BBox Out/1
  Variable Selector/1 -> Centroid Out/1

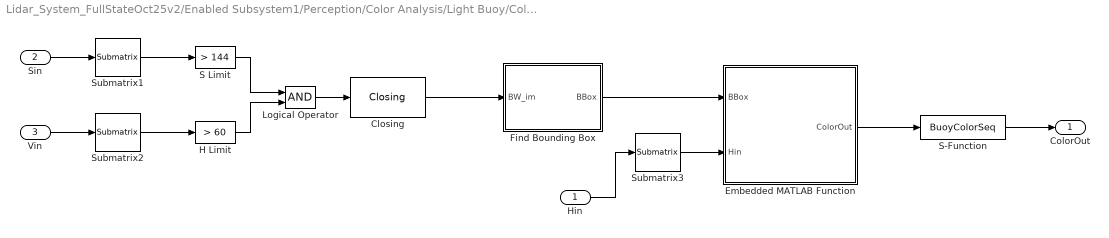
== system Lidar_System_FullStateOct25v2/Enabled Subsystem1/Perception/Color Analysis/Light Buoy/Color Detection ==
  Hin : Inport  OutDataType=fixdt(1, 16)  OutScaling=2^0
  Sin : Inport  Port=2  OutDataType=fixdt(1, 16)  OutScaling=2^0
  Vin : Inport  Port=3  OutDataType=fixdt(1, 16)  OutScaling=2^0
  Closing : vipmorphops/Closing  nhoodsrc=Specify via dialog  strel=strel('square',10)
  Embedded MATLAB Function : Stateflow chart
  Find Bounding Box : Subsystem
  H Limit : simulink/Logic and Bit Operations/Compare To Constant  SystemSampleTime=-1  relop=>  const=60  LogicOutDataTypeMode=uint8  ZeroCross=off
  Logical Operator : Logic  AllPortsSameDT=off  OutDataTypeMode=boolean  LogicDataType=fixdt(0, 8)  OutDataTypeStr=boolean
  S Limit : simulink/Logic and Bit Operations/Compare To Constant  SystemSampleTime=-1  relop=>  const=144  LogicOutDataTypeMode=uint8  ZeroCross=off
  S-Function : S-Function  FunctionName=BuoyColorSeq  EnableBusSupport=off
  Submatrix1 : dspmtrx3/Submatrix  RowSpan=Range of rows  RowStartMode=Index  RowStartIndex=75  RowEndMode=Index  RowEndIndex=225  ColSpan=Range of columns  ColStartMode=Index  ColStartIndex=40  ColEndMode=Index  ColEndIndex=640
  Submatrix2 : dspmtrx3/Submatrix  RowSpan=Range of rows  RowStartMode=Index  RowStartIndex=75  RowEndMode=Index  RowEndIndex=225  ColSpan=Range of columns  ColStartMode=Index  ColStartIndex=40  ColEndMode=Index  ColEndIndex=640
  Submatrix3 : dspmtrx3/Submatrix  RowSpan=Range of rows  RowStartMode=Index  RowStartIndex=75  RowEndMode=Index  RowEndIndex=225  ColSpan=Range of columns  ColStartMode=Index  ColStartIndex=40  ColEndMode=Index  ColEndIndex=640
  ColorOut : Outport  OutDataType=fixdt(1, 16)  OutScaling=2^0
  wires:
  S-Function/1 -> ColorOut/1
  Embedded MATLAB Function/1(ColorOut) -> S-Function/1
  Hin/1 -> Submatrix3/1
  Find Bounding Box/1(BBox) -> Embedded MATLAB Function/1(BBox)
  Closing/1 -> Find Bounding Box/1(BW_im)
  Logical Operator/1 -> Closing/1
  H Limit/1 -> Logical Operator/2
  S Limit/1 -> Logical Operator/1
  Vin/1 -> Submatrix2/1
  Sin/1 -> Submatrix1/1
  Submatrix1/1 -> S Limit/1
  Submatrix2/1 -> H Limit/1
  Submatrix3/1 -> Embedded MATLAB Function/2(Hin)

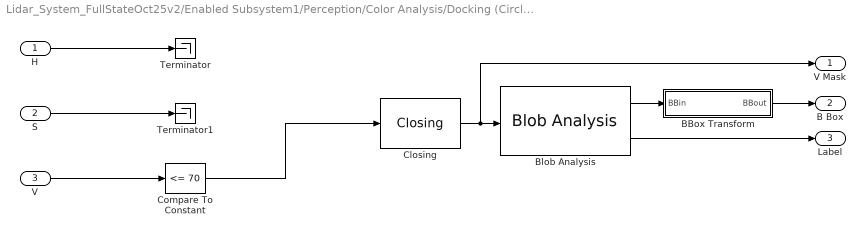
== system Lidar_System_FullStateOct25v2/Enabled Subsystem1/Perception/Color Analysis/Docking (Circle)/Docking1/Blob Analysis ==
  H : Inport  OutDataType=fixdt(1, 16)  OutScaling=2^0
  S : Inport  Port=2  OutDataType=fixdt(1, 16)  OutScaling=2^0
  V : Inport  Port=3  OutDataType=fixdt(1, 16)  OutScaling=2^0
  BBox Transform : Stateflow chart
  Blob Analysis : vipstatistics/Blob Analysis  DialogController=vipDDGCreate  DialogControllerArgs=DataTag0  area=off  centroid=off  bBox=on  majorAxis=off  minorAxis=off  angle=off  eccentricity=off  equivDiameterSq=off  extent=off  perimeter=off  maxBlobs=10  warnIfNumBlobsExceeded=on  isCount=off  useMinArea=on  minArea=400  useMaxArea=off  maxArea=intmax('uint32')  excludeBorderBlob=on  outDT=double  isOutVarDim=off  isFill=on  fillValues=-1  conn=8  isLabel=on  outputMode=Binary point scaling  outputWordLength=32  outputFracLength=16  firstCoeffMode=Binary point scaling  firstCoeffWordLength=16  firstCoeffFracLength=14  secondCoeffMode=Binary point scaling  secondCoeffWordLength=32  secondCoeffFracLength=16  accumMode=Binary point scaling  accumWordLength=32  accumFracLength=0  prodOutputMode=Binary point scaling  prodOutputWordLength=32  prodOutputFracLength=16  roundingMode=Floor  overflowMode=off
  Closing : vipmorphops/Closing  nhoodsrc=Specify via dialog  strel=strel('disk',1,8)
  Compare To Constant : simulink/Logic and Bit Operations/Compare To Constant  SystemSampleTime=-1  relop=<=  const=70  LogicOutDataTypeMode=boolean  ZeroCross=off
  Terminator : Terminator
  Terminator1 : Terminator
  V Mask : Outport  OutDataType=fixdt(1, 16)  OutScaling=2^0
  B Box : Outport  Port=2  OutDataType=fixdt(1, 16)  OutScaling=2^0
  Label : Outport  Port=3  OutDataType=fixdt(1, 16)  OutScaling=2^0
  wires:
  Blob Analysis/2 -> Label/1
  Blob Analysis/1 -> BBox Transform/1(BBin)
  Closing/1 -> Blob Analysis/1, V Mask/1
  BBox Transform/1(BBout) -> B Box/1
  V/1 -> Compare To Constant/1
  S/1 -> Terminator1/1
  H/1 -> Terminator/1
  Compare To Constant/1 -> Closing/1

== system Lidar_System_FullStateOct25v2/Enabled Subsystem1/Perception/Color Analysis/Docking (Circle)/Docking1/Detection ==
  Parametes : Inport  OutDataType=fixdt(1, 16)  OutScaling=2^0
  V Mask : Inport  Port=2  OutDataType=fixdt(1, 16)  OutScaling=2^0
  BBox In : Inport  Port=3  OutDataType=fixdt(1, 16)  OutScaling=2^0
  Label : Inport  Port=4  OutDataType=fixdt(1, 16)  OutScaling=2^0
  Bus Selector : BusSelector  OutputSignals=Templates.Cruciform,Templates.Circle,Templates.Triangle,White Pix Count,Threshold
  Detection : Stateflow chart
  Subsystem : Subsystem
  BBox Out : Outport  OutDataType=fixdt(1, 16)  OutScaling=2^0
  wires:
  Parametes/1 -> Bus Selector/1
  Bus Selector/1 -> Detection/1(cruciform)  "<Cruciform>"
  Bus Selector/2 -> Detection/2(circle)  "<Circle>"
  Bus Selector/3 -> Detection/3(triangle)  "<Triangle>"
  Bus Selector/4 -> Detection/4(whitePixCount)  "<White Pix Count>"
  Bus Selector/5 -> Detection/5(threshold)  "<Threshold>"
  V Mask/1 -> Detection/6(V_mask)
  BBox In/1 -> Detection/7(bbox_in)
  Label/1 -> Detection/8(label)
  Detection/2(rtnRatioDiff) -> Subsystem/2(Idx)
  Detection/1(bbox_out) -> Subsystem/1(BBox in)
  Subsystem/1(BBox out) -> BBox Out/1

== system Lidar_System_FullStateOct25v2/Enabled Subsystem1/Perception/Color Analysis/Docking (Circle)/Docking1/Parameters ==
  Target : Inport
  Bus Creator : BusCreator
  Ratio Difference Threshold : Constant  Value=0.6  OutDataType=fixdt(1, 16)  OutScaling=2^0
  Templates : Subsystem
  White Pixel Count : Constant  Value="[144\t64\t180]"  OutDataType=fixdt(1, 16)  OutScaling=2^0
  Parameters : Outport  OutDataType=fixdt(1, 16)  OutScaling=2^0
  wires:
  Target/1 -> Bus Creator/1  "Target Template"
  Templates/1(Templates) -> Bus Creator/2  "Templates"
  White Pixel Count/1 -> Bus Creator/3  "White Pix Count"
  Ratio Difference Threshold/1 -> Bus Creator/4  "Threshold"
  Bus Creator/1 -> Parameters/1

== system Lidar_System_FullStateOct25v2/Enabled Subsystem1/Perception/Color Analysis/Docking (Circle)/Docking1/Recognition ==
  Parametes : Inport  OutDataType=fixdt(1, 16)  OutScaling=2^0
  BBox In : Inport  Port=2  OutDataType=fixdt(1, 16)  OutScaling=2^0
  V Mask : Inport  Port=3  OutDataType=fixdt(1, 16)  OutScaling=2^0
  Bus Selector : BusSelector  OutputSignals=Target Template,Templates.Cruciform,Templates.Circle,Templates.Triangle,White Pix Count,Threshold
  Embedded MATLAB Function : Stateflow chart
  Subsystem : Subsystem
  BBox Out : Outport  OutDataType=fixdt(1, 16)  OutScaling=2^0
  wires:
  Subsystem/1(BBox out) -> BBox Out/1
  Parametes/1 -> Bus Selector/1
  Bus Selector/1 -> Embedded MATLAB Function/1(targetTemp)  "<Target Template>"
  Bus Selector/2 -> Embedded MATLAB Function/2(cruciform)  "<Cruciform>"
  Bus Selector/3 -> Embedded MATLAB Function/3(circle)  "<Circle>"
  Bus Selector/4 -> Embedded MATLAB Function/4(triangle)  "<Triangle>"
  Bus Selector/5 -> Embedded MATLAB Function/5(whitePixCount)  "<White Pix Count>"
  Bus Selector/6 -> Embedded MATLAB Function/6(threshold)  "<Threshold>"
  V Mask/1 -> Embedded MATLAB Function/7(V_mask)
  BBox In/1 -> Embedded MATLAB Function/8(bbox_in)
  Embedded MATLAB Function/1(bbox_out) -> Subsystem/1(BBox in)
  Embedded MATLAB Function/2(returnRatioDiff) -> Subsystem/2(Idx)

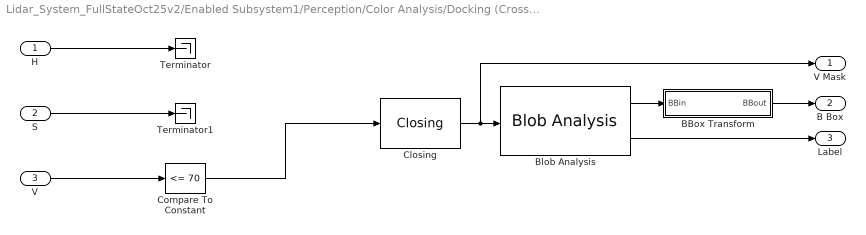
== system Lidar_System_FullStateOct25v2/Enabled Subsystem1/Perception/Color Analysis/Docking (Cross)/Docking1/Blob Analysis ==
  H : Inport  OutDataType=fixdt(1, 16)  OutScaling=2^0
  S : Inport  Port=2  OutDataType=fixdt(1, 16)  OutScaling=2^0
  V : Inport  Port=3  OutDataType=fixdt(1, 16)  OutScaling=2^0
  BBox Transform : Stateflow chart
  Blob Analysis : vipstatistics/Blob Analysis  DialogController=vipDDGCreate  DialogControllerArgs=DataTag4  area=off  centroid=off  bBox=on  majorAxis=off  minorAxis=off  angle=off  eccentricity=off  equivDiameterSq=off  extent=off  perimeter=off  maxBlobs=10  warnIfNumBlobsExceeded=on  isCount=off  useMinArea=on  minArea=400  useMaxArea=off  maxArea=intmax('uint32')  excludeBorderBlob=on  outDT=double  isOutVarDim=off  isFill=on  fillValues=-1  conn=8  isLabel=on  outputMode=Binary point scaling  outputWordLength=32  outputFracLength=16  firstCoeffMode=Binary point scaling  firstCoeffWordLength=16  firstCoeffFracLength=14  secondCoeffMode=Binary point scaling  secondCoeffWordLength=32  secondCoeffFracLength=16  accumMode=Binary point scaling  accumWordLength=32  accumFracLength=0  prodOutputMode=Binary point scaling  prodOutputWordLength=32  prodOutputFracLength=16  roundingMode=Floor  overflowMode=off
  Closing : vipmorphops/Closing  nhoodsrc=Specify via dialog  strel=strel('disk',1,8)
  Compare To Constant : simulink/Logic and Bit Operations/Compare To Constant  SystemSampleTime=-1  relop=<=  const=70  LogicOutDataTypeMode=boolean  ZeroCross=off
  Terminator : Terminator
  Terminator1 : Terminator
  V Mask : Outport  OutDataType=fixdt(1, 16)  OutScaling=2^0
  B Box : Outport  Port=2  OutDataType=fixdt(1, 16)  OutScaling=2^0
  Label : Outport  Port=3  OutDataType=fixdt(1, 16)  OutScaling=2^0
  wires:
  Compare To Constant/1 -> Closing/1
  H/1 -> Terminator/1
  S/1 -> Terminator1/1
  V/1 -> Compare To Constant/1
  BBox Transform/1(BBout) -> B Box/1
  Closing/1 -> V Mask/1, Blob Analysis/1
  Blob Analysis/1 -> BBox Transform/1(BBin)
  Blob Analysis/2 -> Label/1

== system Lidar_System_FullStateOct25v2/Enabled Subsystem1/Perception/Color Analysis/Docking (Cross)/Docking1/Detection ==
  Parametes : Inport  OutDataType=fixdt(1, 16)  OutScaling=2^0
  V Mask : Inport  Port=2  OutDataType=fixdt(1, 16)  OutScaling=2^0
  BBox In : Inport  Port=3  OutDataType=fixdt(1, 16)  OutScaling=2^0
  Label : Inport  Port=4  OutDataType=fixdt(1, 16)  OutScaling=2^0
  Bus Selector : BusSelector  OutputSignals=Templates.Cruciform,Templates.Circle,Templates.Triangle,White Pix Count,Threshold
  Detection : Stateflow chart
  Subsystem : Subsystem
  BBox Out : Outport  OutDataType=fixdt(1, 16)  OutScaling=2^0
  wires:
  Subsystem/1(BBox out) -> BBox Out/1
  Detection/1(bbox_out) -> Subsystem/1(BBox in)
  Detection/2(rtnRatioDiff) -> Subsystem/2(Idx)
  Label/1 -> Detection/8(label)
  BBox In/1 -> Detection/7(bbox_in)
  V Mask/1 -> Detection/6(V_mask)
  Bus Selector/5 -> Detection/5(threshold)  "<Threshold>"
  Bus Selector/4 -> Detection/4(whitePixCount)  "<White Pix Count>"
  Bus Selector/3 -> Detection/3(triangle)  "<Triangle>"
  Bus Selector/2 -> Detection/2(circle)  "<Circle>"
  Bus Selector/1 -> Detection/1(cruciform)  "<Cruciform>"
  Parametes/1 -> Bus Selector/1

== system Lidar_System_FullStateOct25v2/Enabled Subsystem1/Perception/Color Analysis/Docking (Cross)/Docking1/Parameters ==
  Target : Inport
  Bus Creator : BusCreator
  Ratio Difference Threshold : Constant  Value=0.6  OutDataType=fixdt(1, 16)  OutScaling=2^0
  Templates : Subsystem
  White Pixel Count : Constant  Value="[144\t64\t180]"  OutDataType=fixdt(1, 16)  OutScaling=2^0
  Parameters : Outport  OutDataType=fixdt(1, 16)  OutScaling=2^0
  wires:
  Bus Creator/1 -> Parameters/1
  Ratio Difference Threshold/1 -> Bus Creator/4  "Threshold"
  White Pixel Count/1 -> Bus Creator/3  "White Pix Count"
  Templates/1(Templates) -> Bus Creator/2  "Templates"
  Target/1 -> Bus Creator/1  "Target Template"

== system Lidar_System_FullStateOct25v2/Enabled Subsystem1/Perception/Color Analysis/Docking (Cross)/Docking1/Recognition ==
  Parametes : Inport  OutDataType=fixdt(1, 16)  OutScaling=2^0
  BBox In : Inport  Port=2  OutDataType=fixdt(1, 16)  OutScaling=2^0
  V Mask : Inport  Port=3  OutDataType=fixdt(1, 16)  OutScaling=2^0
  Bus Selector : BusSelector  OutputSignals=Target Template,Templates.Cruciform,Templates.Circle,Templates.Triangle,White Pix Count,Threshold
  Embedded MATLAB Function : Stateflow chart
  Subsystem : Subsystem
  BBox Out : Outport  OutDataType=fixdt(1, 16)  OutScaling=2^0
  wires:
  Embedded MATLAB Function/2(returnRatioDiff) -> Subsystem/2(Idx)
  Embedded MATLAB Function/1(bbox_out) -> Subsystem/1(BBox in)
  BBox In/1 -> Embedded MATLAB Function/8(bbox_in)
  V Mask/1 -> Embedded MATLAB Function/7(V_mask)
  Bus Selector/6 -> Embedded MATLAB Function/6(threshold)  "<Threshold>"
  Bus Selector/5 -> Embedded MATLAB Function/5(whitePixCount)  "<White Pix Count>"
  Bus Selector/4 -> Embedded MATLAB Function/4(triangle)  "<Triangle>"
  Bus Selector/3 -> Embedded MATLAB Function/3(circle)  "<Circle>"
  Bus Selector/2 -> Embedded MATLAB Function/2(cruciform)  "<Cruciform>"
  Bus Selector/1 -> Embedded MATLAB Function/1(targetTemp)  "<Target Template>"
  Parametes/1 -> Bus Selector/1
  Subsystem/1(BBox out) -> BBox Out/1

== system Lidar_System_FullStateOct25v2/Enabled Subsystem1/Perception/Color Analysis/Docking (Triangle)/Docking1/Blob Analysis ==
  H : Inport  OutDataType=fixdt(1, 16)  OutScaling=2^0
  S : Inport  Port=2  OutDataType=fixdt(1, 16)  OutScaling=2^0
  V : Inport  Port=3  OutDataType=fixdt(1, 16)  OutScaling=2^0
  BBox Transform : Stateflow chart
  Blob Analysis : vipstatistics/Blob Analysis  DialogController=vipDDGCreate  DialogControllerArgs=DataTag8  area=off  centroid=off  bBox=on  majorAxis=off  minorAxis=off  angle=off  eccentricity=off  equivDiameterSq=off  extent=off  perimeter=off  maxBlobs=10  warnIfNumBlobsExceeded=on  isCount=off  useMinArea=on  minArea=400  useMaxArea=off  maxArea=intmax('uint32')  excludeBorderBlob=on  outDT=double  isOutVarDim=off  isFill=on  fillValues=-1  conn=8  isLabel=on  outputMode=Binary point scaling  outputWordLength=32  outputFracLength=16  firstCoeffMode=Binary point scaling  firstCoeffWordLength=16  firstCoeffFracLength=14  secondCoeffMode=Binary point scaling  secondCoeffWordLength=32  secondCoeffFracLength=16  accumMode=Binary point scaling  accumWordLength=32  accumFracLength=0  prodOutputMode=Binary point scaling  prodOutputWordLength=32  prodOutputFracLength=16  roundingMode=Floor  overflowMode=off
  Closing : vipmorphops/Closing  nhoodsrc=Specify via dialog  strel=strel('disk',1,8)
  Compare To Constant : simulink/Logic and Bit Operations/Compare To Constant  SystemSampleTime=-1  relop=<=  const=70  LogicOutDataTypeMode=boolean  ZeroCross=off
  Terminator : Terminator
  Terminator1 : Terminator
  V Mask : Outport  OutDataType=fixdt(1, 16)  OutScaling=2^0
  B Box : Outport  Port=2  OutDataType=fixdt(1, 16)  OutScaling=2^0
  Label : Outport  Port=3  OutDataType=fixdt(1, 16)  OutScaling=2^0
  wires:
  Compare To Constant/1 -> Closing/1
  H/1 -> Terminator/1
  S/1 -> Terminator1/1
  V/1 -> Compare To Constant/1
  BBox Transform/1(BBout) -> B Box/1
  Closing/1 -> V Mask/1, Blob Analysis/1
  Blob Analysis/1 -> BBox Transform/1(BBin)
  Blob Analysis/2 -> Label/1

== system Lidar_System_FullStateOct25v2/Enabled Subsystem1/Perception/Color Analysis/Docking (Triangle)/Docking1/Detection ==
  Parametes : Inport  OutDataType=fixdt(1, 16)  OutScaling=2^0
  V Mask : Inport  Port=2  OutDataType=fixdt(1, 16)  OutScaling=2^0
  BBox In : Inport  Port=3  OutDataType=fixdt(1, 16)  OutScaling=2^0
  Label : Inport  Port=4  OutDataType=fixdt(1, 16)  OutScaling=2^0
  Bus Selector : BusSelector  OutputSignals=Templates.Cruciform,Templates.Circle,Templates.Triangle,White Pix Count,Threshold
  Detection : Stateflow chart
  Subsystem : Subsystem
  BBox Out : Outport  OutDataType=fixdt(1, 16)  OutScaling=2^0
  wires:
  Subsystem/1(BBox out) -> BBox Out/1
  Detection/1(bbox_out) -> Subsystem/1(BBox in)
  Detection/2(rtnRatioDiff) -> Subsystem/2(Idx)
  Label/1 -> Detection/8(label)
  BBox In/1 -> Detection/7(bbox_in)
  V Mask/1 -> Detection/6(V_mask)
  Bus Selector/5 -> Detection/5(threshold)  "<Threshold>"
  Bus Selector/4 -> Detection/4(whitePixCount)  "<White Pix Count>"
  Bus Selector/3 -> Detection/3(triangle)  "<Triangle>"
  Bus Selector/2 -> Detection/2(circle)  "<Circle>"
  Bus Selector/1 -> Detection/1(cruciform)  "<Cruciform>"
  Parametes/1 -> Bus Selector/1

== system Lidar_System_FullStateOct25v2/Enabled Subsystem1/Perception/Color Analysis/Docking (Triangle)/Docking1/Parameters ==
  Target : Inport
  Bus Creator : BusCreator
  Ratio Difference Threshold : Constant  Value=0.6  OutDataType=fixdt(1, 16)  OutScaling=2^0
  Templates : Subsystem
  White Pixel Count : Constant  Value="[144\t64\t180]"  OutDataType=fixdt(1, 16)  OutScaling=2^0
  Parameters : Outport  OutDataType=fixdt(1, 16)  OutScaling=2^0
  wires:
  Bus Creator/1 -> Parameters/1
  Ratio Difference Threshold/1 -> Bus Creator/4  "Threshold"
  White Pixel Count/1 -> Bus Creator/3  "White Pix Count"
  Templates/1(Templates) -> Bus Creator/2  "Templates"
  Target/1 -> Bus Creator/1  "Target Template"

== system Lidar_System_FullStateOct25v2/Enabled Subsystem1/Perception/Color Analysis/Docking (Triangle)/Docking1/Recognition ==
  Parametes : Inport  OutDataType=fixdt(1, 16)  OutScaling=2^0
  BBox In : Inport  Port=2  OutDataType=fixdt(1, 16)  OutScaling=2^0
  V Mask : Inport  Port=3  OutDataType=fixdt(1, 16)  OutScaling=2^0
  Bus Selector : BusSelector  OutputSignals=Target Template,Templates.Cruciform,Templates.Circle,Templates.Triangle,White Pix Count,Threshold
  Embedded MATLAB Function : Stateflow chart
  Subsystem : Subsystem
  BBox Out : Outport  OutDataType=fixdt(1, 16)  OutScaling=2^0
  wires:
  Embedded MATLAB Function/2(returnRatioDiff) -> Subsystem/2(Idx)
  Embedded MATLAB Function/1(bbox_out) -> Subsystem/1(BBox in)
  BBox In/1 -> Embedded MATLAB Function/8(bbox_in)
  V Mask/1 -> Embedded MATLAB Function/7(V_mask)
  Bus Selector/6 -> Embedded MATLAB Function/6(threshold)  "<Threshold>"
  Bus Selector/5 -> Embedded MATLAB Function/5(whitePixCount)  "<White Pix Count>"
  Bus Selector/4 -> Embedded MATLAB Function/4(triangle)  "<Triangle>"
  Bus Selector/3 -> Embedded MATLAB Function/3(circle)  "<Circle>"
  Bus Selector/2 -> Embedded MATLAB Function/2(cruciform)  "<Cruciform>"
  Bus Selector/1 -> Embedded MATLAB Function/1(targetTemp)  "<Target Template>"
  Parametes/1 -> Bus Selector/1
  Subsystem/1(BBox out) -> BBox Out/1
